simulink model "BUCKS"  (R2022b)
settings: Solver=VariableStepAuto  StartTime=0.0  StopTime=1  RelTol=1e-3
undefined symbols (not defined in the file or in its folder): C, L, R, U
settings Model: Creator=fermo  LastModifiedBy=fermo

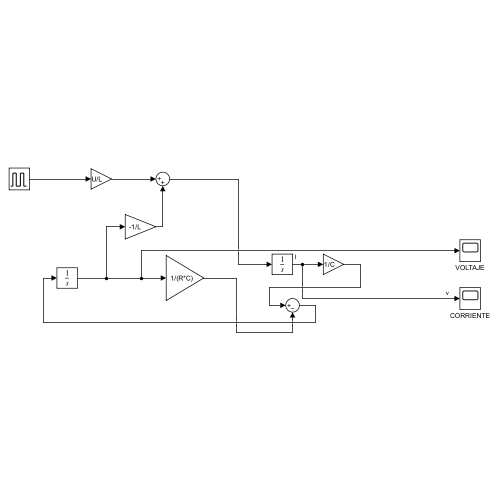
[thumbnail: Simulink's stored preview of the top-level diagram]
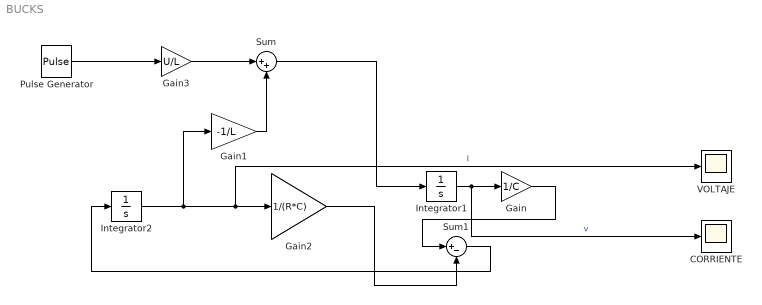
== system BUCKS ==
  CORRIENTE : Scope
  Gain : Gain  Gain=1/C
  Gain1 : Gain  Gain=-1/L
  Gain2 : Gain  Gain=1/(R*C)
  Gain3 : Gain  Gain=U/L
  Integrator1 : Integrator
  Integrator2 : Integrator
  Pulse Generator : DiscretePulseGenerator  PulseType=Time based  Period=0.00001  PulseWidth=40
  Sum : Sum  Inputs=|++
  Sum1 : Sum  Inputs=|+-
  VOLTAJE : Scope
  wires:
  Pulse Generator/1 -> Gain3/1
  Gain3/1 -> Sum/1
  Gain1/1 -> Sum/2
  Integrator2/1 -> Gain1/1, VOLTAJE/1, Gain2/1  "I"
  Integrator1/1 -> CORRIENTE/1, Gain/1  "v"
  Gain2/1 -> Sum1/2
  Gain/1 -> Sum1/1
  Sum1/1 -> Integrator2/1
  Sum/1 -> Integrator1/1
